simulink model "LinearADPSimullink_R2015a"  (R2018b)
settings: Solver=ode45  StartTime=0.0  StopTime=10  MaxStep=0.0001  RelTol=1e-3  EnableMultiTasking=on
undefined symbols (not defined in the file): rank
libraries: simulink x3
settings Model: Creator=Yuri  LastModifiedBy=KyThuat88
settings SolverCC: ZeroCrossControl=EnableAll  ZeroCrossAlgorithm=Adaptive
settings DataIOCC: LimitDataPoints=on  SaveFormat=Array
settings OptimizationCC: LifeSpan=inf
settings DebuggingCC: AlgebraicLoopMsg=none  SolverPrmCheckMsg=warning  MultiTaskDSMMsg=none  SFUnexpectedBacktrackingDiag=warning  SFNoUnconditionalDefaultTransitionDiag=warning  SFExecutionAtInitializationDiag=none
settings HardwareCC: ProdBitPerPointer=32  ProdBitPerSizeT=32  ProdBitPerPtrDiffT=32  ProdLargestAtomicFloat=None  ProdIntDivRoundTo=Undefined  ProdEndianess=Unspecified  ProdWordSize=32  ProdHWDeviceType=32-bit Generic
settings ModelReferenceCC: PropagateSignalLabelsOutOfModel=off
settings SFSimCC: SimUseLocalCustomCode=off
settings RTWCC: GenCodeOnly=on  RTWUseLocalCustomCode=off
settings CodeAppCC: StateflowObjectComments=on
settings GRTTargetCC: TargetLangStandard=C89/C90 (ANSI)  GeneratePreprocessorConditionals=Disable all
settings ConfigComp: CovMetricSettings=dw  CovHtmlReporting=on  CovSaveCumulativeToWorkspaceVar=on  CovSaveSingleToWorkspaceVar=on  CovExternalEMLEnable=off  CovSFcnEnable=off

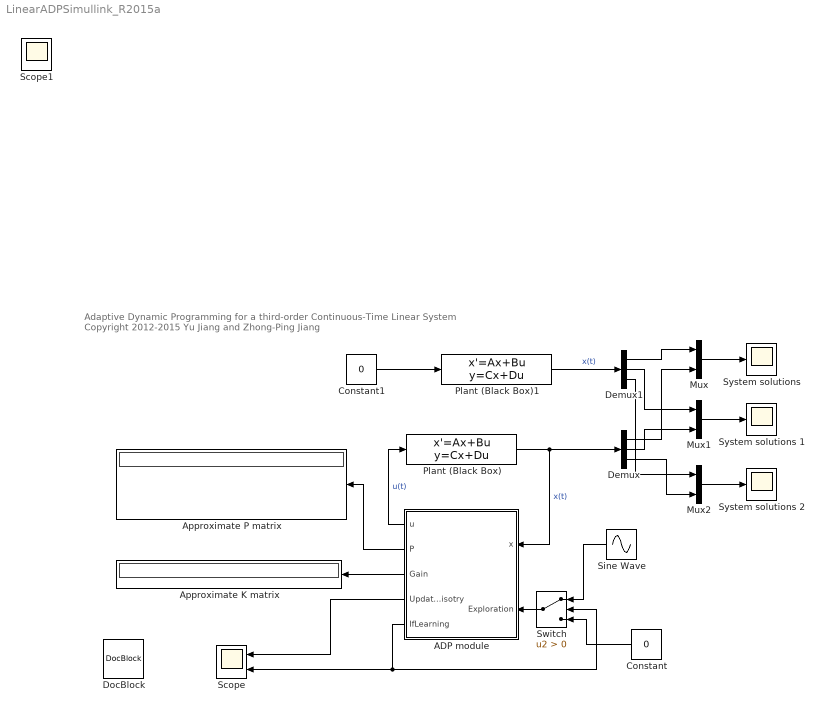
== system LinearADPSimullink_R2015a ==
  note: Adaptive Dynamic Programming for a third-order Continuous-Time Linear System
      |
      | Copyright 2012-2015 Yu Jiang and Zhong-Ping Jiang
  ADP module : Subsystem  mask{K=[0,0,0], Q=eye(3), R=1, dT=0.1, epsilon=.0005}
      mask prompts: K "Initial Gain K (e.g., [0,0])"; Q "Weight Matrix Q (e.g., eye(2))"; R "Weight R (e.g., 1)"; dT "Linearning Interval dT (e.g., 0.01)"; epsilon "Threshold (e.g., 0.00001)"
  Approximate K matrix : Display
  Approximate P matrix : Display
  Constant : Constant  Value=0
  Constant1 : Constant  Value=0
  Demux : Demux  Outputs=3
  Demux1 : Demux  Outputs=3
  DocBlock : simulink/Model-Wide Utilities/DocBlock  DocumentType=Text
      content=|
      | %To verify the results, try:
      |
      | A = [0 1 0; 0 0 1;-0.1 -0.5 -0.7];
      | B = [0;0;1];
      | Q = eye(3);
      | R = 1;
      |
      | [Popt,~,Kopt] = care(A,B,Q,R)
  Mux : Mux  Inputs=2
  Mux1 : Mux  Inputs=2
  Mux2 : Mux  Inputs=2
  Plant (Black Box) : StateSpace  A=[0 1 0; 0 0 1;-0.1 -0.5 -0.7]  B=[0;0;1]  C=eye(3)  D=zeros(3,1)  InitialCondition=[10;-10;15]
  Plant (Black Box)1 : StateSpace  A=[0 1 0; 0 0 1;-0.1 -0.5 -0.7]  B=[0;0;1]  C=eye(3)  D=zeros(3,1)  InitialCondition=[10;-10;15]
  Scope : Scope  NumInputPorts=2
  Sine Wave : Sin  Amplitude=2  Frequency=10  SampleTime=0.0001
  Switch : Switch  Criteria=u2 > Threshold  SampleTime=0.0001
  "System solutions " : Scope
  System solutions 1 : Scope
  System solutions 2 : Scope
  Scope1 : Scope
  wires:
  Plant (Black Box)/1 -> Demux/1, ADP module/1(x)  "x(t)"
  ADP module/1(u) -> Plant (Black Box)/1  "u(t)"
  ADP module/2("P ") -> Approximate P matrix/1
  ADP module/3(Gain) -> Approximate K matrix/1
  ADP module/4(UpdateHisotry) -> Scope/1
  Sine Wave/1 -> Switch/1
  Switch/1 -> ADP module/2(Exploration)
  Constant/1 -> Switch/3
  Constant1/1 -> Plant (Black Box)1/1
  Plant (Black Box)1/1 -> Demux1/1  "x(t)"
  Demux1/1 -> Mux/1
  Demux/1 -> Mux/2
  Mux/1 -> "System solutions "/1
  Demux1/2 -> Mux1/1
  Demux/2 -> Mux1/2
  Demux1/3 -> Mux2/1
  Demux/3 -> Mux2/2
  Mux1/1 -> System solutions 1/1
  Mux2/1 -> System solutions 2/1
  ADP module/5(IfLearning) -> Scope/2, Switch/2

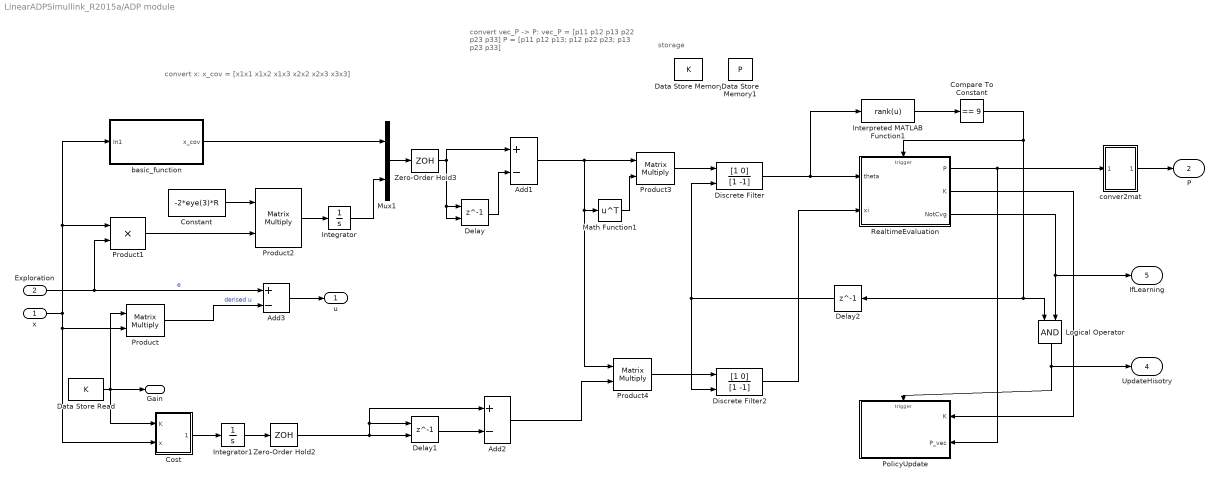
== system LinearADPSimullink_R2015a/ADP module ==
  note: convert x:
      | x_cov = [x1x1 x1x2 x1x3 x2x2 x2x3 x3x3]
  note: storage
  note: convert  vec_P -> P:
      |
      | vec_P = [p11 p12 p13 p22 p23 p33]
      |
      | P = [p11 p12 p13;
      |        p12 p22 p23;
      |        p13 p23 p33]
  x : Inport  PortDimensions=3
  Exploration : Inport  Port=2
  Add1 : Sum  Inputs=+-
  Add2 : Sum  Inputs=+-
  Add3 : Sum  Inputs=+-
  Compare To Constant : simulink/Logic and Bit Operations/Compare To Constant  relop===  const=9  OutDataTypeStr=boolean
  Constant : Constant  Value=-2*eye(3)*R  VectorParams1D=off
  Cost : Subsystem
  Data Store Memory : DataStoreMemory  Priority=1  DataStoreName=K  InitialValue=K  VectorParams1D=off  ShowAdditionalParam=off  Dimensions=[1,3]
  Data Store Memory1 : DataStoreMemory  DataStoreName=P  InitialValue=-1*ones(6,1)  ShowAdditionalParam=off
  Data Store Read : DataStoreRead  DataStoreName=K  SampleTime=0
  Delay : Delay  DelayLength=1  InitialConditionSource=Input port  InitialCondition=0  SampleTime=dT
      settings: InputPortMap=u0,p4
  Delay1 : Delay  DelayLength=1  InitialConditionSource=Input port  InitialCondition=0  SampleTime=dT
      settings: InputPortMap=u0,p4
  Delay2 : Delay  DelayLength=1  InitialCondition=0  SampleTime=dT
  Discrete Filter : DiscreteFilter  Numerator=[1 0]  Denominator=[1 -1]  ExternalReset=Rising  FilterStructure=Direct form I  SampleTime=dT  NumAccumDataTypeStr=Inherit: Same as product output  OutDataTypeStr=Inherit: Same as input
      settings: InputPortMap=u0,r7
  Discrete Filter2 : DiscreteFilter  Numerator=[1 0]  Denominator=[1 -1]  ExternalReset=Rising  FilterStructure=Direct form I  SampleTime=dT  NumAccumDataTypeStr=Inherit: Same as product output  OutDataTypeStr=Inherit: Same as input
      settings: InputPortMap=u0,r7
  Integrator : Integrator
  Integrator1 : Integrator
  Interpreted MATLAB Function1 : MATLABFcn  MATLABFcn=rank(u)
  Logical Operator : Logic  AllPortsSameDT=off  OutDataTypeStr=boolean
  Math Function1 : Math  Operator=transpose  SaturateOnIntegerOverflow=on
  Mux1 : Mux  Inputs=2
  PolicyUpdate : Subsystem
  Product{,2..4} (4 alike) : Product  Multiplication=Matrix(*)
  Product1 : Product
  RealtimeEvaluation : Subsystem
  Zero-Order Hold2 : ZeroOrderHold  SampleTime=dT
  Zero-Order Hold3 : ZeroOrderHold  SampleTime=dT
  basic_function : Subsystem
  conver2mat : Subsystem
  u : Outport
  "P " : Outport  Port=2
  Gain : Outport  Port=3
  UpdateHisotry : Outport  Port=4
  IfLearning : Outport  Port=5
  wires:
  RealtimeEvaluation/3(NotCvg) -> Logical Operator/2, IfLearning/1
  Exploration/1 -> Product1/2, Add3/1  "e"
  Logical Operator/1 -> PolicyUpdate/Trigger, UpdateHisotry/1
  Compare To Constant/1 -> Delay2/1, Logical Operator/1, RealtimeEvaluation/Trigger
  Add1/1 -> Product3/1, Math Function1/1, Product4/1
  Delay2/1 -> Discrete Filter2/2, Discrete Filter/2
  Zero-Order Hold2/1 -> Add2/1, Delay1/1, Delay1/2
  Mux1/1 -> Zero-Order Hold3/1
  Discrete Filter2/1 -> RealtimeEvaluation/2(xi)
  Discrete Filter/1 -> Interpreted MATLAB Function1/1, RealtimeEvaluation/1(theta)
  Product4/1 -> Discrete Filter2/1
  Add2/1 -> Product4/2
  Product3/1 -> Discrete Filter/1
  Math Function1/1 -> Product3/2
  Add3/1 -> u/1
  Delay1/1 -> Add2/2
  Integrator1/1 -> Zero-Order Hold2/1
  Cost/1(r(x,uk)) -> Integrator1/1
  Delay/1 -> Add1/2
  Zero-Order Hold3/1 -> Add1/1, Delay/1, Delay/2
  Integrator/1 -> Mux1/2
  Product2/1 -> Integrator/1
  Constant/1 -> Product2/1
  Product1/1 -> Product2/2
  Data Store Read/1 -> Product/1, Gain/1, Cost/1(K)
  Product/1 -> Add3/2  "derised u"
  x/1 -> basic_function/1(In1), Product1/1, Product/2, Cost/2(x)
  RealtimeEvaluation/1(P) -> PolicyUpdate/2("P_vec "), conver2mat/1(In1)
  RealtimeEvaluation/2(K) -> PolicyUpdate/1(K)
  Interpreted MATLAB Function1/1 -> Compare To Constant/1
  basic_function/1(x_cov) -> Mux1/1
  conver2mat/1(Out1) -> "P "/1

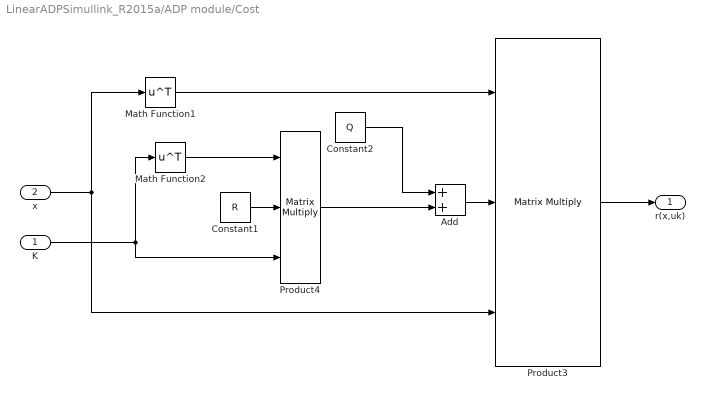
== system LinearADPSimullink_R2015a/ADP module/Cost ==
  K : Inport
  x : Inport  Port=2  PortDimensions=3
  Add : Sum
  Constant1 : Constant  Value=R
  Constant2 : Constant  Value=Q
  Math Function1 : Math  Operator=transpose  SaturateOnIntegerOverflow=on
  Math Function2 : Math  Operator=transpose  SaturateOnIntegerOverflow=on
  Product3 : Product  Inputs=3  Multiplication=Matrix(*)
  Product4 : Product  Inputs=3  Multiplication=Matrix(*)
  r(x,uk) : Outport
  wires:
  Math Function2/1 -> Product4/1
  Constant1/1 -> Product4/2
  K/1 -> Product4/3, Math Function2/1
  Constant2/1 -> Add/1
  Product3/1 -> r(x,uk)/1
  Math Function1/1 -> Product3/1
  Product4/1 -> Add/2
  x/1 -> Product3/3, Math Function1/1
  Add/1 -> Product3/2

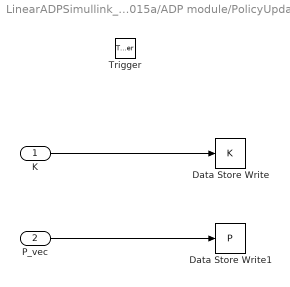
== system LinearADPSimullink_R2015a/ADP module/PolicyUpdate ==
  K : Inport  OutDataTypeStr=double  PortDimensions=[1,3]
  "P_vec " : Inport  Port=2  PortDimensions=6
  Trigger : TriggerPort  VariantControl=(inherit)  OutputDataType=double  PortDimensions=1
  Data Store Write : DataStoreWrite  DataStoreName=K
  Data Store Write1 : DataStoreWrite  DataStoreName=P
  wires:
  "P_vec "/1 -> Data Store Write1/1
  K/1 -> Data Store Write/1

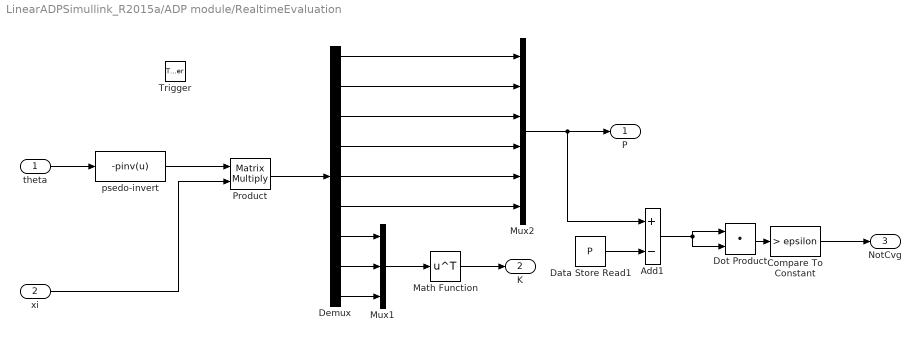
== system LinearADPSimullink_R2015a/ADP module/RealtimeEvaluation ==
  theta : Inport
  xi : Inport  Port=2
  Trigger : TriggerPort  VariantControl=(inherit)  OutputDataType=double  PortDimensions=1
  Add1 : Sum  Inputs=+-
  Compare To Constant : simulink/Logic and Bit Operations/Compare To Constant  relop=>  const=epsilon  OutDataTypeStr=boolean
  Data Store Read1 : DataStoreRead  DataStoreName=P
  Demux : Demux  Outputs=9
  Dot Product : DotProduct  InputSameDT=on  OutDataTypeStr=Inherit: Inherit via internal rule
  Math Function : Math  Operator=transpose  SaturateOnIntegerOverflow=on
  Mux1 : Mux  Inputs=3
  Mux2 : Mux  Inputs=6
  Product : Product  Multiplication=Matrix(*)  OutDataTypeStr=double
  psedo-invert : MATLABFcn  MATLABFcn=-pinv(u)  Output1D=off
  P : Outport  OutDataTypeStr=double  PortDimensions=6  InitialOutput=zeros(6,1)
  K : Outport  Port=2  PortDimensions=[1,3]  InitialOutput=K
  NotCvg : Outport  Port=3  PortDimensions=1  InitialOutput=1
  wires:
  Compare To Constant/1 -> NotCvg/1
  Mux2/1 -> Add1/1, P/1
  Dot Product/1 -> Compare To Constant/1
  Add1/1 -> Dot Product/1, Dot Product/2
  Data Store Read1/1 -> Add1/2
  Product/1 -> Demux/1
  theta/1 -> psedo-invert/1
  xi/1 -> Product/2
  Math Function/1 -> K/1
  Mux1/1 -> Math Function/1
  Demux/7 -> Mux1/1
  Demux/8 -> Mux1/2
  Demux/9 -> Mux1/3
  Demux/1 -> Mux2/1
  Demux/2 -> Mux2/2
  Demux/3 -> Mux2/3
  Demux/4 -> Mux2/4
  Demux/5 -> Mux2/5
  Demux/6 -> Mux2/6
  psedo-invert/1 -> Product/1

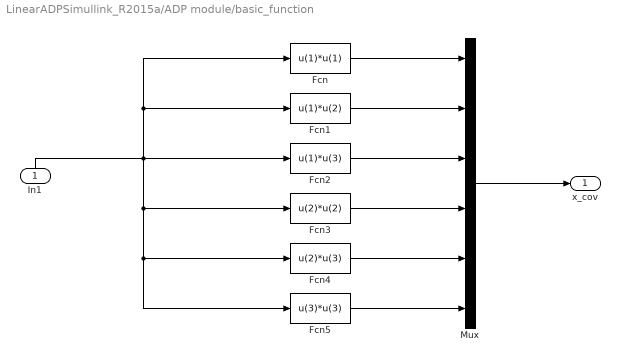
== system LinearADPSimullink_R2015a/ADP module/basic_function ==
  In1 : Inport
  Fcn : Fcn  Expr=u(1)*u(1)
  Fcn1 : Fcn  Expr=u(1)*u(2)
  Fcn2 : Fcn  Expr=u(1)*u(3)
  Fcn3 : Fcn  Expr=u(2)*u(2)
  Fcn4 : Fcn  Expr=u(2)*u(3)
  Fcn5 : Fcn  Expr=u(3)*u(3)
  Mux : Mux  Inputs=6
  x_cov : Outport  PortDimensions=6
  wires:
  Mux/1 -> x_cov/1
  In1/1 -> Fcn2/1, Fcn/1, Fcn1/1, Fcn3/1, Fcn5/1, Fcn4/1
  Fcn3/1 -> Mux/4
  Fcn4/1 -> Mux/5
  Fcn5/1 -> Mux/6
  Fcn1/1 -> Mux/2
  Fcn2/1 -> Mux/3
  Fcn/1 -> Mux/1

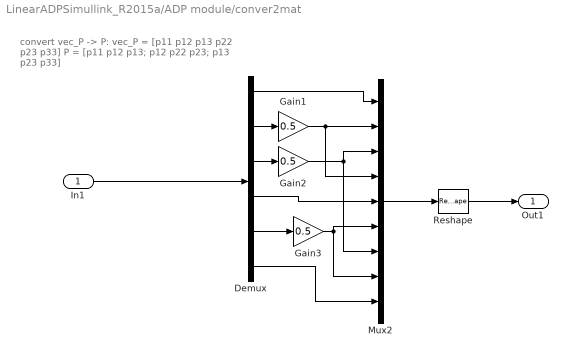
== system LinearADPSimullink_R2015a/ADP module/conver2mat ==
  note: convert  vec_P -> P:
      |
      | vec_P = [p11 p12 p13 p22 p23 p33]
      |
      | P = [p11 p12 p13;
      |        p12 p22 p23;
      |        p13 p23 p33]
  In1 : Inport
  Demux : Demux  Outputs=6
  Gain1 : Gain  Gain=0.5
  Gain2 : Gain  Gain=0.5
  Gain3 : Gain  Gain=0.5
  Mux2 : Mux  Inputs=9
  Reshape : Reshape  OutputDimensionality=Customize  OutputDimensions=[3,3]
  Out1 : Outport
  wires:
  In1/1 -> Demux/1
  Demux/2 -> Gain1/1
  Demux/3 -> Gain2/1
  Mux2/1 -> Reshape/1
  Gain3/1 -> Mux2/8, Mux2/6
  Reshape/1 -> Out1/1
  Demux/5 -> Gain3/1
  Gain2/1 -> Mux2/7, Mux2/3
  Gain1/1 -> Mux2/4, Mux2/2
  Demux/1 -> Mux2/1
  Demux/4 -> Mux2/5
  Demux/6 -> Mux2/9
